simulink model "Non_Isolated_Cuk_Converter"  (R2021a)
settings: Solver=VariableStepAuto  StartTime=0.0  StopTime=0.1  RelTol=1e-3
libraries: spsSeriesRLCBranchLib x5, spsCurrentMeasurementLib x5, spsVoltageMeasurementLib x4, spsDiodeLib x1, spsMosfetLib x1, spsDCVoltageSourceLib x1, spspowerguiLib x1
settings Model: Creator=EREN-PC  LastModifiedBy=EREN-PC

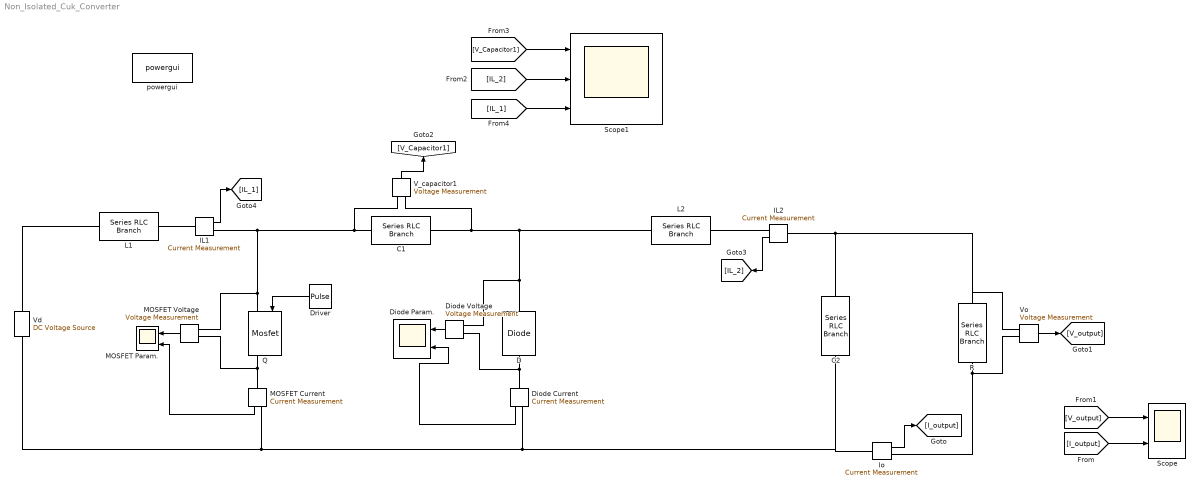
== system Non_Isolated_Cuk_Converter ==
  C1 : spsSeriesRLCBranchLib/Series RLC Branch  LConnTagsString=__new0  RConnTagsString=__new0  BranchType=C  Resistance=1  Inductance=1e-3  SetiL0=off  InitialCurrent=0  Capacitance=180e-6  Setx0=off  InitialVoltage=0  Measurements=None
  C2 : spsSeriesRLCBranchLib/Series RLC Branch  LConnTagsString=__new0  RConnTagsString=__new0  BranchType=C  Resistance=1  Inductance=1e-3  SetiL0=off  InitialCurrent=0  Capacitance=20e-6  Setx0=off  InitialVoltage=0  Measurements=None
  D : spsDiodeLib/Diode  Ron=0.001  Lon=0  Vf=0.8  IC=0  UseSnubber=0  Rs=500  Cs=250e-9  Measurements=off
  Diode Current : spsCurrentMeasurementLib/Current Measurement  PhasorSimulation=off  OutputType=Complex  PSBequivalent=0
  Diode Param. : Scope  NumInputPorts=2
  Diode Voltage : spsVoltageMeasurementLib/Voltage Measurement  PhasorSimulation=off  OutputType=Complex  PSBequivalent=0
  Driver : DiscretePulseGenerator  PulseType=Time based  Period=1/50000  PulseWidth=45
  IL1 : spsCurrentMeasurementLib/Current Measurement  PhasorSimulation=off  OutputType=Complex  PSBequivalent=0
  IL2 : spsCurrentMeasurementLib/Current Measurement  PhasorSimulation=off  OutputType=Complex  PSBequivalent=0
  Io : spsCurrentMeasurementLib/Current Measurement  PhasorSimulation=off  OutputType=Complex  PSBequivalent=0
  L1 : spsSeriesRLCBranchLib/Series RLC Branch  LConnTagsString=__new0  RConnTagsString=__new0  BranchType=L  Resistance=1  Inductance=2.2e-3  SetiL0=off  InitialCurrent=0  Capacitance=1e-6  Setx0=off  InitialVoltage=0  Measurements=None
  L2 : spsSeriesRLCBranchLib/Series RLC Branch  LConnTagsString=__new0  RConnTagsString=__new0  BranchType=L  Resistance=1  Inductance=2.2e-3  SetiL0=off  InitialCurrent=0  Capacitance=1e-6  Setx0=off  InitialVoltage=0  Measurements=None
  MOSFET Current : spsCurrentMeasurementLib/Current Measurement  PhasorSimulation=off  OutputType=Complex  PSBequivalent=0
  MOSFET Param. : Scope  NumInputPorts=2
  MOSFET Voltage : spsVoltageMeasurementLib/Voltage Measurement  PhasorSimulation=off  OutputType=Complex  PSBequivalent=0
  Q : spsMosfetLib/Mosfet  Ron=0.1  Lon=0  Rd=0.01  Vfd=0  IC=0  Rs=1e5  Cs=inf  Measurements=on
  R : spsSeriesRLCBranchLib/Series RLC Branch  LConnTagsString=__new0  RConnTagsString=__new0  BranchType=R  Resistance=6  Inductance=1e-3  SetiL0=off  InitialCurrent=0  Capacitance=1e-6  Setx0=off  InitialVoltage=0  Measurements=None
  Scope : Scope  NumInputPorts=2
  Scope1 : Scope  NumInputPorts=3
  V_capacitor1 : spsVoltageMeasurementLib/Voltage Measurement  PhasorSimulation=off  OutputType=Complex  PSBequivalent=0
  Vd : spsDCVoltageSourceLib/DC Voltage Source  Amplitude=16  Measurements=None
  Vo : spsVoltageMeasurementLib/Voltage Measurement  PhasorSimulation=off  OutputType=Complex  PSBequivalent=0
  powergui : spspowerguiLib/powergui  Priority=1  SimulationMode=Continuous  SampleTime=50e-6  frequency=60  Iterations=50  frequencyindice=0  Pbase=100e6  ErrMax=1e-4  UnitsV=kV  UnitsW=MW  buscounter=0  FunctionMessages=off  echomessages=off  EnableUseOfTLC=off  CurrentSourceSwitches=off  DisableSnubberDevices=off  DisableRonSwitches=off  DisableVfSwitches=off  DisplayEquations=off  AutomaticDiscreteSolvers=off  SolverType=Tustin/Backward Euler (TBE)  Interpol=off  ExternalGateDelay=off  methode=off  Ts=100  x0status=blocks  SPID=on  SwTol=0  HookPort=off  NonlinearTolerance=1e-4  nMaxIteration=100  ContinueOnMaxIteration=off  RestoreLinks=warning  ResistiveCurrentMeasurement=off  Frange=[0:2:500]  Ylog=off  Xlog=on  ShowGrid=off  save=off  variable=ZData  structure=0  ZoomFFT=off  StartTime=0.0  cycles=1  DisplayStyle=1  fundamental=60  FreqAxis=off  MaxFrequency=1000  frequencyindicesteady=1  RmsSteady=1  display=off
  wires:
  Driver/1 -> Q/1
  Io/1 -> [I_output]
  Vo/1 -> [V_output]
  [V_output] -> Scope/1
  [I_output] -> Scope/2
  V_capacitor1/1 -> [V_Capacitor1]
  IL2/1 -> [IL_2]
  [V_Capacitor1] -> Scope1/1
  [IL_2] -> Scope1/2
  IL1/1 -> [IL_1]
  [IL_1] -> Scope1/3
  MOSFET Current/1 -> MOSFET Param./2
  MOSFET Voltage/1 -> MOSFET Param./1
  Diode Current/1 -> Diode Param./2
  Diode Voltage/1 -> Diode Param./1
  connections:
  Vd/RConn1 -- L1/LConn1
  C1/LConn1 -- MOSFET Voltage/LConn1 -- Q/LConn1 -- IL1/RConn1 -- V_capacitor1/LConn1
  C2/LConn1 -- Io/LConn1 -- Diode Current/RConn1 -- Vd/LConn1 -- MOSFET Current/RConn1
  D/LConn1 -- Diode Voltage/LConn1 -- V_capacitor1/LConn2 -- C1/RConn1 -- L2/RConn1
  R/LConn1 -- Io/RConn1 -- Vo/LConn1
  IL2/RConn1 -- L2/LConn1
  C2/RConn1 -- Vo/LConn2 -- R/RConn1 -- IL2/LConn1
  IL1/LConn1 -- L1/RConn1
  Q/RConn1 -- MOSFET Current/LConn1 -- MOSFET Voltage/LConn2
  D/RConn1 -- Diode Current/LConn1 -- Diode Voltage/LConn2
